simulink model "Test_Encoder_64_to_6_Low_Word"  (Simulink 8.7)
settings: Solver=ode45  StartTime=0.0  StopTime=len  RelTol=1e-3
libraries: commutil2 x2, Encoders_Lib x1, Miscellaneous x1
settings Model: Creator=N  LastModifiedBy=Jozko Mrkvicka
settings DataIOCC: LimitDataPoints=off
settings DebuggingCC: UnderspecifiedInitializationDetection=Simplified  MergeDetectMultiDrivingBlocksExec=error
settings HardwareCC: ProdBitPerPointer=64  ProdLargestAtomicFloat=Float  ProdIntDivRoundTo=Zero  ProdEndianess=LittleEndian  ProdHWDeviceType=Intel->x86-64 (Windows64)
settings ModelReferenceCC: PropagateSignalLabelsOutOfModel=on

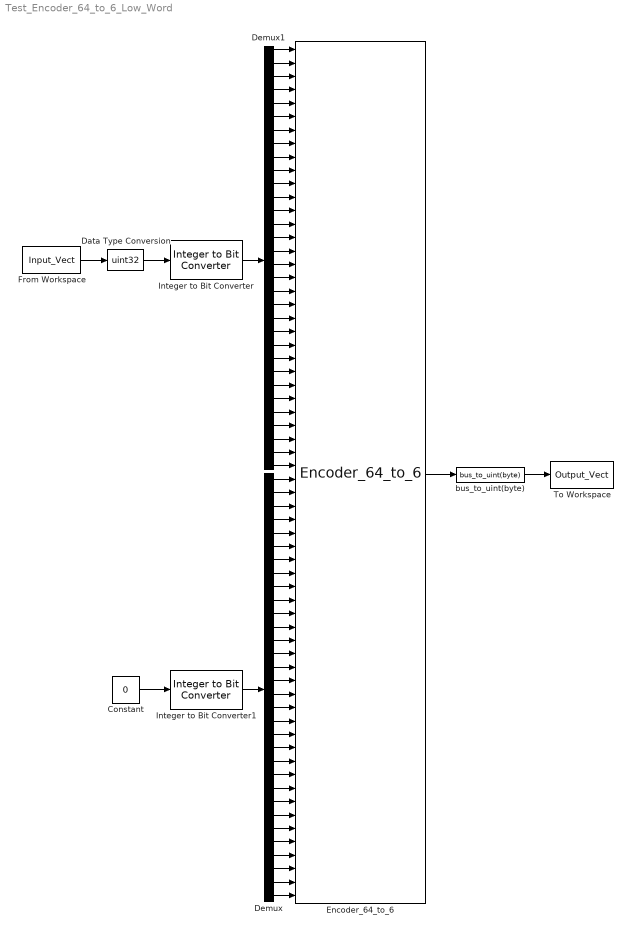
== system Test_Encoder_64_to_6_Low_Word ==
  Constant : Constant  Value=0  OutDataTypeStr=uint32
  Data Type Conversion : DataTypeConversion  OutDataTypeStr=uint32
  Demux : Demux  Outputs=32
  Demux1 : Demux  Outputs=32
  Encoder_64_to_6 : Encoders_Lib/Encoders_Lib/Encoder_64_to_6
  From Workspace : FromWorkspace  VariableName=Input_Vect  SampleTime=1  Interpolate=off  OutputAfterFinalValue=Holding final value
  Integer to Bit Converter : commutil2/Integer to Bit Converter  nbits=32  signedInputValues=Unsigned  bitOrder=MSB first  outDtype=boolean
  Integer to Bit Converter1 : commutil2/Integer to Bit Converter  nbits=32  signedInputValues=Unsigned  bitOrder=MSB first  outDtype=boolean
  To Workspace : ToWorkspace  VariableName=Output_Vect  SampleTime=1
  bus_to_uint(byte) : Miscellaneous/bus_to_uint(byte)
  wires:
  Encoder_64_to_6/1 -> bus_to_uint(byte)/1
  bus_to_uint(byte)/1 -> To Workspace/1
  Demux/1 -> Encoder_64_to_6/33
  Demux/2 -> Encoder_64_to_6/34
  Demux/3 -> Encoder_64_to_6/35
  Demux/4 -> Encoder_64_to_6/36
  Demux/5 -> Encoder_64_to_6/37
  Demux/6 -> Encoder_64_to_6/38
  Demux/7 -> Encoder_64_to_6/39
  Demux/8 -> Encoder_64_to_6/40
  Demux/9 -> Encoder_64_to_6/41
  Demux/10 -> Encoder_64_to_6/42
  Demux/11 -> Encoder_64_to_6/43
  Demux/12 -> Encoder_64_to_6/44
  Demux/13 -> Encoder_64_to_6/45
  Demux/14 -> Encoder_64_to_6/46
  Demux/15 -> Encoder_64_to_6/47
  Demux/16 -> Encoder_64_to_6/48
  Demux/17 -> Encoder_64_to_6/49
  Demux/18 -> Encoder_64_to_6/50
  Demux/19 -> Encoder_64_to_6/51
  Demux/20 -> Encoder_64_to_6/52
  Demux/21 -> Encoder_64_to_6/53
  Demux/22 -> Encoder_64_to_6/54
  Demux/23 -> Encoder_64_to_6/55
  Demux/24 -> Encoder_64_to_6/56
  Demux/25 -> Encoder_64_to_6/57
  Demux/26 -> Encoder_64_to_6/58
  Demux/27 -> Encoder_64_to_6/59
  Demux/28 -> Encoder_64_to_6/60
  Demux/29 -> Encoder_64_to_6/61
  Demux/30 -> Encoder_64_to_6/62
  Demux/31 -> Encoder_64_to_6/63
  Demux/32 -> Encoder_64_to_6/64
  Demux1/1 -> Encoder_64_to_6/1
  Demux1/2 -> Encoder_64_to_6/2
  Demux1/3 -> Encoder_64_to_6/3
  Demux1/4 -> Encoder_64_to_6/4
  Demux1/5 -> Encoder_64_to_6/5
  Demux1/6 -> Encoder_64_to_6/6
  Demux1/7 -> Encoder_64_to_6/7
  Demux1/8 -> Encoder_64_to_6/8
  Demux1/9 -> Encoder_64_to_6/9
  Demux1/10 -> Encoder_64_to_6/10
  Demux1/11 -> Encoder_64_to_6/11
  Demux1/12 -> Encoder_64_to_6/12
  Demux1/13 -> Encoder_64_to_6/13
  Demux1/14 -> Encoder_64_to_6/14
  Demux1/15 -> Encoder_64_to_6/15
  Demux1/16 -> Encoder_64_to_6/16
  Demux1/17 -> Encoder_64_to_6/17
  Demux1/18 -> Encoder_64_to_6/18
  Demux1/19 -> Encoder_64_to_6/19
  Demux1/20 -> Encoder_64_to_6/20
  Demux1/21 -> Encoder_64_to_6/21
  Demux1/22 -> Encoder_64_to_6/22
  Demux1/23 -> Encoder_64_to_6/23
  Demux1/24 -> Encoder_64_to_6/24
  Demux1/25 -> Encoder_64_to_6/25
  Demux1/26 -> Encoder_64_to_6/26
  Demux1/27 -> Encoder_64_to_6/27
  Demux1/28 -> Encoder_64_to_6/28
  Demux1/29 -> Encoder_64_to_6/29
  Demux1/30 -> Encoder_64_to_6/30
  Demux1/31 -> Encoder_64_to_6/31
  Demux1/32 -> Encoder_64_to_6/32
  Integer to Bit Converter/1 -> Demux1/1
  Data Type Conversion/1 -> Integer to Bit Converter/1
  From Workspace/1 -> Data Type Conversion/1
  Integer to Bit Converter1/1 -> Demux/1
  Constant/1 -> Integer to Bit Converter1/1
